simulink model "inner_pid_discrete_grant"  (R2019a)
settings: Solver=VariableStepAuto  StartTime=0.0  StopTime=60  RelTol=1e-3  EnableMultiTasking=on
undefined symbols (not defined in the file or in its folder): b, feedforward_thrust, inner_h, inner_maxlim, inner_minlim, k, l
libraries: cstblocks x1

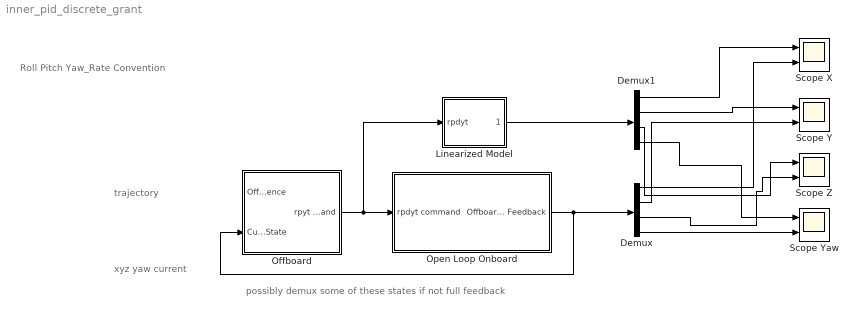
== system inner_pid_discrete_grant ==
  note: trajectory
  note: xyz yaw current
  note: possibly demux some of these states if not full feedback
  note: Roll Pitch Yaw_Rate Convention
  Demux : Demux
  Demux1 : Demux
  Linearized Model : Subsystem
  Offboard : Subsystem
  Open Loop Onboard : Subsystem
  "Scope X " : Scope  NumInputPorts=2
  Scope Y : Scope  NumInputPorts=2
  Scope Yaw : Scope  NumInputPorts=2
  Scope Z : Scope  NumInputPorts=2
  wires:
  ? -> Offboard/1("Offboard Reference ")
  Offboard/1(rpyt command) -> Linearized Model/1(rpdyt), Open Loop Onboard/1(rpdyt command)
  Open Loop Onboard/1(Offboard Feedback) -> Offboard/2("Current State "), Demux/1
  Demux1/1 -> "Scope X "/1
  Demux/1 -> "Scope X "/2
  Demux1/2 -> Scope Y/1
  Demux/2 -> Scope Y/2
  Demux1/3 -> Scope Z/1
  Demux/3 -> Scope Z/2
  Demux1/4 -> Scope Yaw/1
  Demux/4 -> Scope Yaw/2
  Linearized Model/1(xyzyaw) -> Demux1/1

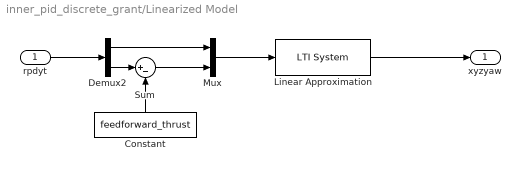
== system inner_pid_discrete_grant/Linearized Model ==
  rpdyt : Inport
  Constant : Constant  Value=feedforward_thrust
  Demux2 : Demux  Outputs=[3 1]
  Linear Approximation : cstblocks/LTI System  sys=linsys1  IC=[]
  Mux : Mux  Inputs=[3 1]
  Sum : Sum  Inputs=|+-
  xyzyaw : Outport
  wires:
  Demux2/1 -> Mux/1
  Sum/1 -> Mux/2
  rpdyt/1 -> Demux2/1
  Demux2/2 -> Sum/1
  Linear Approximation/1 -> xyzyaw/1
  Mux/1 -> Linear Approximation/1
  Constant/1 -> Sum/2

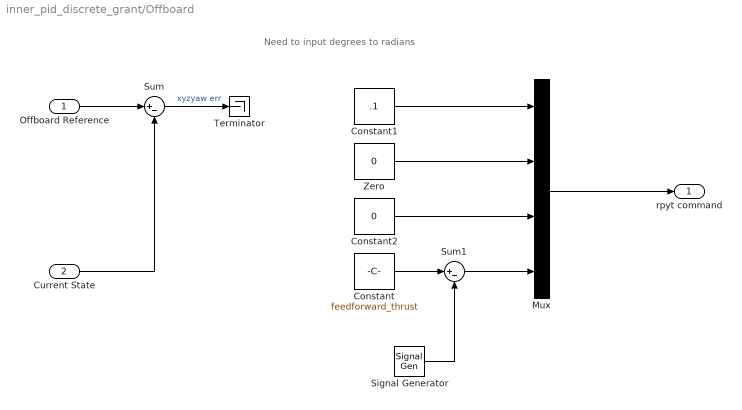
== system inner_pid_discrete_grant/Offboard ==
  note: Need to input degrees to radians
  "Offboard Reference " : Inport
  "Current State " : Inport  Port=2
  Constant : Constant  Value=feedforward_thrust
  Constant1 : Constant  Value=.1
  Constant2 : Constant  Value=0
  Mux : Mux
  Signal Generator : SignalGenerator  Amplitude=10000  Units=rad/sec
  Sum : Sum  Inputs=|+-
  Sum1 : Sum  Inputs=|+-
  Terminator : Terminator
  Zero : Constant  Value=0  OutDataTypeStr=Inherit: Inherit via back propagation
  rpyt command : Outport
  wires:
  Mux/1 -> rpyt command/1
  Zero/1 -> Mux/2
  Constant1/1 -> Mux/1
  Constant2/1 -> Mux/3
  "Current State "/1 -> Sum/2
  "Offboard Reference "/1 -> Sum/1
  Sum/1 -> Terminator/1  "xyzyaw err"
  Signal Generator/1 -> Sum1/2
  Sum1/1 -> Mux/4
  Constant/1 -> Sum1/1

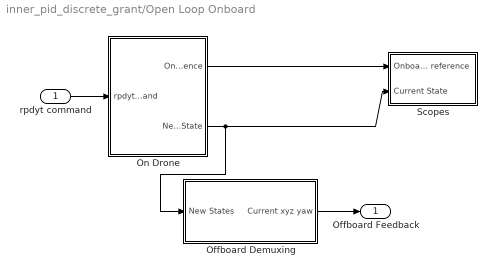
== system inner_pid_discrete_grant/Open Loop Onboard ==
  rpdyt command : Inport
  Offboard Demuxing : Subsystem
  On Drone : Subsystem
  Scopes : Subsystem
  Offboard Feedback : Outport
  wires:
  rpdyt command/1 -> On Drone/1(rpdyt command)
  On Drone/2(New State) -> Scopes/2(Current State), Offboard Demuxing/1(New States)
  On Drone/1(Onboard Reference) -> Scopes/1(Onboard reference)
  Offboard Demuxing/1(Current xyz yaw) -> Offboard Feedback/1

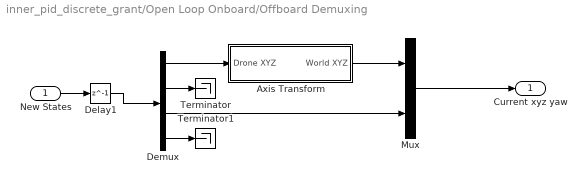
== system inner_pid_discrete_grant/Open Loop Onboard/Offboard Demuxing ==
  New States : Inport
  Axis Transform : Subsystem
  Delay1 : Delay  DelayLength=1  InitialCondition=0  SampleTime=inner_h
  Demux : Demux  Outputs=[3 5 1 3]
  Mux : Mux  Inputs=2
  Terminator : Terminator
  Terminator1 : Terminator
  Current xyz yaw : Outport
  wires:
  Mux/1 -> Current xyz yaw/1
  New States/1 -> Delay1/1
  Delay1/1 -> Demux/1
  Demux/2 -> Terminator/1
  Demux/1 -> Axis Transform/1(Drone XYZ)
  Demux/3 -> Mux/2
  Demux/4 -> Terminator1/1
  Axis Transform/1(World XYZ) -> Mux/1

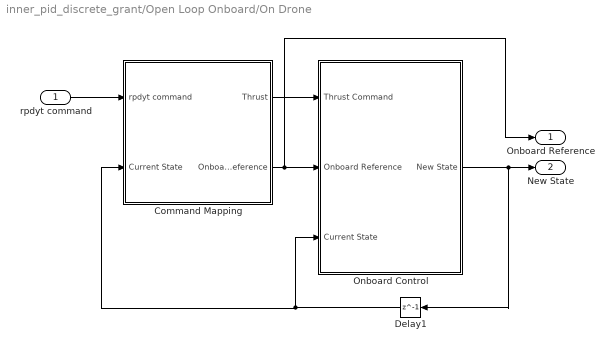
== system inner_pid_discrete_grant/Open Loop Onboard/On Drone ==
  rpdyt command : Inport
  Command Mapping : Subsystem
  Delay1 : Delay  DelayLength=1  InitialCondition=0  SampleTime=inner_h
  "Onboard Control " : Subsystem
  Onboard Reference : Outport
  New State : Outport  Port=2
  wires:
  rpdyt command/1 -> Command Mapping/1(rpdyt command)
  "Onboard Control "/1(New State) -> Delay1/1, New State/1
  Command Mapping/1(Thrust) -> "Onboard Control "/1(Thrust Command)
  Command Mapping/2(Onboard Reference) -> Onboard Reference/1, "Onboard Control "/2(Onboard Reference)
  Delay1/1 -> Command Mapping/2(Current State), "Onboard Control "/3(Current State)

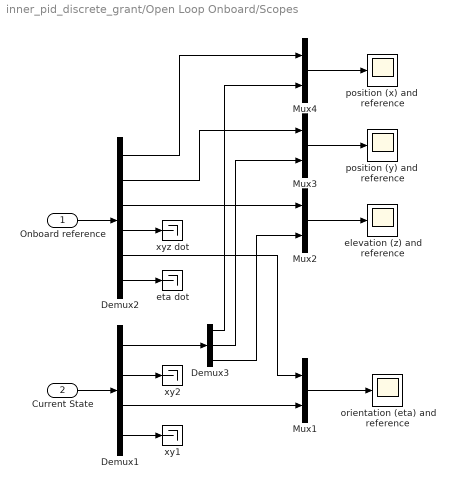
== system inner_pid_discrete_grant/Open Loop Onboard/Scopes ==
  Onboard reference : Inport
  Current State : Inport  Port=2
  "   eta dot" : Terminator
  "   xy1" : Terminator
  "   xy2" : Terminator
  "  xyz dot" : Terminator
  Demux1 : Demux  Outputs=[3,3,3,3]
  Demux2 : Demux  Outputs=[1,1,1,3,3,3]
  Demux3 : Demux  Outputs=[1,1,1]
  Mux{1..4} (4 alike) : Mux  Inputs=2
  elevation (z) and reference : Scope
  orientation (eta) and reference : Scope
  position (x) and  reference : Scope
  position (y) and  reference : Scope
  wires:
  Demux3/3 -> Mux2/2
  Mux1/1 -> orientation (eta) and reference/1
  Mux4/1 -> position (x) and  reference/1
  Demux2/5 -> Mux1/1
  Mux2/1 -> elevation (z) and reference/1
  Demux2/1 -> Mux4/1
  Demux1/3 -> Mux1/2
  Current State/1 -> Demux1/1
  Demux1/4 -> "   xy1"/1
  Demux2/3 -> Mux2/1
  Demux2/4 -> "  xyz dot"/1
  Demux2/2 -> Mux3/1
  Mux3/1 -> position (y) and  reference/1
  Demux2/6 -> "   eta dot"/1
  Onboard reference/1 -> Demux2/1
  Demux3/2 -> Mux3/2
  Demux3/1 -> Mux4/2
  Demux1/1 -> Demux3/1
  Demux1/2 -> "   xy2"/1

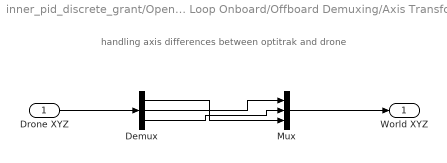
== system inner_pid_discrete_grant/Open Loop Onboard/Offboard Demuxing/Axis Transform ==
  note: handling axis differences between optitrak and drone
  Drone XYZ : Inport
  Demux : Demux  Outputs=3
  Mux : Mux  Inputs=3
  World XYZ : Outport
  wires:
  Drone XYZ/1 -> Demux/1
  Mux/1 -> World XYZ/1
  Demux/1 -> Mux/3
  Demux/2 -> Mux/1
  Demux/3 -> Mux/2

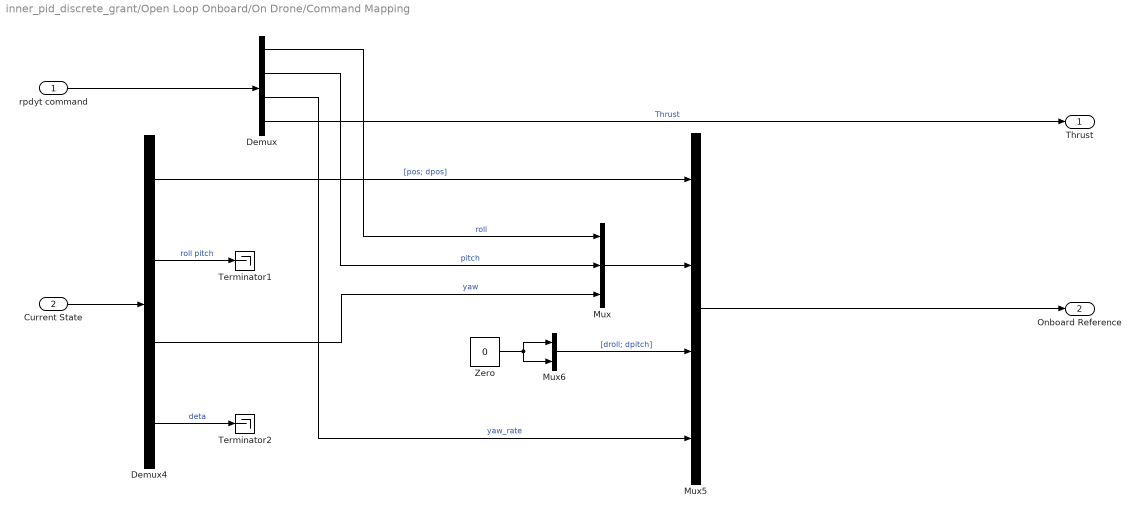
== system inner_pid_discrete_grant/Open Loop Onboard/On Drone/Command Mapping ==
  rpdyt command : Inport
  Current State : Inport  Port=2
  Demux : Demux
  Demux4 : Demux  Outputs=[6 2 1 3]
  Mux : Mux  Inputs=3
  Mux5 : Mux  Inputs=[6 3 2 1]
  Mux6 : Mux  Inputs=2
  Terminator1 : Terminator
  Terminator2 : Terminator
  Zero : Constant  Value=0  OutDataTypeStr=Inherit: Inherit via back propagation
  Thrust : Outport
  Onboard Reference : Outport  Port=2
  wires:
  Demux4/1 -> Mux5/1  "[pos; dpos]"
  Demux4/2 -> Terminator1/1  "roll pitch"
  Demux/4 -> Thrust/1  "Thrust"
  rpdyt command/1 -> Demux/1
  Mux/1 -> Mux5/2
  Current State/1 -> Demux4/1
  Mux6/1 -> Mux5/3  "[droll; dpitch]"
  Demux4/3 -> Mux/3  "yaw"
  Demux4/4 -> Terminator2/1  "deta"
  Demux/1 -> Mux/1  "roll"
  Demux/3 -> Mux5/4  "yaw_rate"
  Mux5/1 -> Onboard Reference/1
  Demux/2 -> Mux/2  "pitch"
  Zero/1 -> Mux6/2, Mux6/1

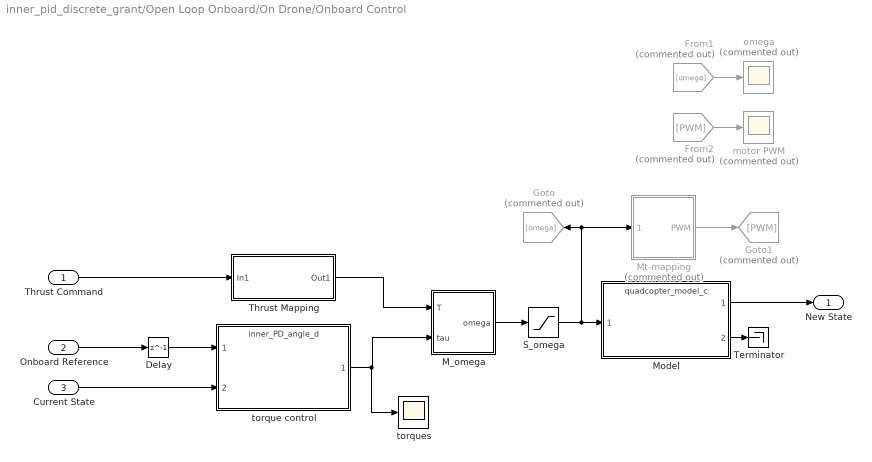
== system inner_pid_discrete_grant/Open Loop Onboard/On Drone/Onboard Control  ==
  Thrust Command : Inport
  Onboard Reference : Inport  Port=2
  Current State : Inport  Port=3
  Delay : Delay  DelayLength=1  InitialCondition=0  SampleTime=inner_h
  From1 : From  Commented=on  GotoTag=omega
  From2 : From  Commented=on  GotoTag=PWM
  Goto : Goto  Commented=on  GotoTag=omega
  Goto1 : Goto  Commented=on  GotoTag=PWM
  M_omega : Subsystem
  Model : ModelReference  ModelNameDialog=quadcopter_model_c.mdl  SimulationMode=Normal  ModelReferenceVersion=1.157
  Mt-mapping : Subsystem  Commented=on
  S_omega : Saturate  UpperLimit=inner_maxlim  LowerLimit=inner_minlim
  Terminator : Terminator
  Thrust Mapping : Subsystem
  motor PWM : Scope  Commented=on
  "omega " : Scope  Commented=on
  torque control : ModelReference  ModelNameDialog=inner_PD_angle_d.slx  SimulationMode=Normal  ModelReferenceVersion=1.86
  torques : Scope
  New State : Outport
  wires:
  Model/2 -> Terminator/1
  torque control/1 -> torques/1, M_omega/2(tau)
  Thrust Mapping/1(Out1) -> M_omega/1(T)
  Mt-mapping/1(PWM) -> Goto1/1
  Onboard Reference/1 -> Delay/1
  Delay/1 -> torque control/1
  Thrust Command/1 -> Thrust Mapping/1(In1)
  S_omega/1 -> Goto/1, Mt-mapping/1(omega), Model/1
  M_omega/1(omega) -> S_omega/1
  Model/1 -> New State/1
  Current State/1 -> torque control/2
  From2/1 -> motor PWM/1
  From1/1 -> "omega "/1

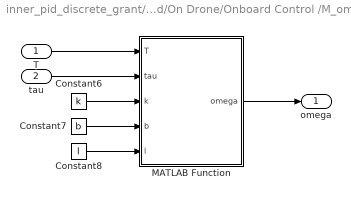
== system inner_pid_discrete_grant/Open Loop Onboard/On Drone/Onboard Control /M_omega ==
  T : Inport
  tau : Inport  Port=2
  Constant6 : Constant  Value=k
  Constant7 : Constant  Value=b
  Constant8 : Constant  Value=l
  MATLAB Function : MATLAB Function  TreatAsAtomicUnit=on
  omega : Outport
  wires:
  Constant7/1 -> MATLAB Function/4(b)
  tau/1 -> MATLAB Function/2(tau)
  Constant6/1 -> MATLAB Function/3(k)
  MATLAB Function/1(omega) -> omega/1
  T/1 -> MATLAB Function/1(T)
  Constant8/1 -> MATLAB Function/5(l)

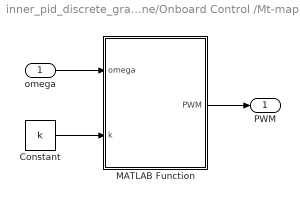
== system inner_pid_discrete_grant/Open Loop Onboard/On Drone/Onboard Control /Mt-mapping ==
  omega : Inport
  Constant : Constant  Value=k
  MATLAB Function : MATLAB Function  TreatAsAtomicUnit=on
  PWM : Outport
  wires:
  MATLAB Function/1(PWM) -> PWM/1
  omega/1 -> MATLAB Function/1(omega)
  Constant/1 -> MATLAB Function/2(k)

== system inner_pid_discrete_grant/Open Loop Onboard/On Drone/Onboard Control /Thrust Mapping ==
  In1 : Inport
  MATLAB Function : MATLAB Function  TreatAsAtomicUnit=on
  Out1 : Outport
  wires:
  In1/1 -> MATLAB Function/1(thrust_in)
  MATLAB Function/1(thrust_out) -> Out1/1

== matlab function inner_pid_discrete_grant/Open Loop Onboard/On Drone/Onboard Control /Thrust Mapping/MATLAB Function ==
function thrust_out  = thrust_mapping(thrust_in)
thrust_out = 9.66418e-6*thrust_in - .0966418;
end

== matlab function inner_pid_discrete_grant/Open Loop Onboard/On Drone/Onboard Control /M_omega/MATLAB Function ==
function omega = Mw(T, tau, k, b, l)
%#codegen
tau_phi = tau(1);
tau_theta = tau(2);
tau_psi = tau(3);
w1sq = T/(4*k) - tau_theta/(2*k*l) - tau_psi / (4*b);
w2sq = T/(4*k) - tau_phi/(2*k*l) + tau_psi / (4*b);
w3sq = T/(4*k) + tau_theta/(2*k*l) - tau_psi / (4*b);
w4sq = T/(4*k) + tau_phi/(2*k*l) + tau_psi / (4*b);

omega = sqrt(max([w1sq w2sq w3sq w4sq]', 0));

== matlab function inner_pid_discrete_grant/Open Loop Onboard/On Drone/Onboard Control /Mt-mapping/MATLAB Function ==
function PWM = Mt(omega, k)
%#codegen
rotor_thrusts = k.*omega.^2;
beta1 = 0.0877;
beta2 = 0.0660;
PWM =  -beta1/(2*beta2) + sqrt((beta1/(2*beta2))^2 + rotor_thrusts/beta2);
